simulink model "Copy_of_eCS_Algo_Simulation_2015b"  (R2015b)
settings: Solver=ode1  StartTime=0.0  StopTime=3  FixedStep=1/80000  RelTol=1e-3
PreLoadFcn:
  | if exist('tl_preloadfcn','file'), tl_preloadfcn(gcs,402); end
PostLoadFcn:
  | , if any(exist('dsrtsu_mdlpostloadfcn', 'file') == [2, 3, 6]), try dsrtsu_mdlpostloadfcn('Execute', bdroot); catch fprintf('Error in PostLoadFcn (dsrtsu_mdlpostloadfcn) for model "%s":\n %s\n', bdroot, lasterr); end, end,
  | if exist('tl_postloadfcn','file'), tl_postloadfcn(gcs,402); end
InitFcn:
  | if exist('tlds_init','file'), tlds_init(gcs); end
StartFcn:
  | if exist('tlds_start','file'), tlds_start(gcs); end
StopFcn:
  | if exist('tlds_stop','file'), tlds_stop(gcs); end
model workspace (MAT data in the model file):
  au8PrevExecProfile = [0 0 0 0 0 0]
values from neighbouring files (symbols this model uses):
  AccSensor = 5    [Parameter_eCS_Algo.m]
  AlgoType = 0    [Parameter_eCS_Algo.m]
  Cxy = 1*0.017    (= 0.017)    [Acc_Init_SelV1.m]
  Cxz = 1*0.017    (= 0.017)    [Acc_Init_SelV1.m]
  Cyx = 1*0.017    (= 0.017)    [Acc_Init_SelV1.m]
  Cyz = 1*0.017    (= 0.017)    [Acc_Init_SelV1.m]
  Czx = 1*0.017    (= 0.017)    [Acc_Init_SelV1.m]
  Czy = 1*0.017    (= 0.017)    [Acc_Init_SelV1.m]
  Forced_Oscillation = 0    [Parameter_eCS_Algo.m]    (also in run_Rotation_sim.m = run)
  FreqTemperature = 10    [Acc_Init_SelV1.m]
  MaxSensorOffset = 0.3    [Acc_Init_SelV1.m]
  Mean_x_noise = 4e-3    (= 0.004)    [Acc_Init_SelV1.m]
  Mean_y_noise = 4e-3    (= 0.004)    [Acc_Init_SelV1.m]
  Mean_z_noise = 4e-3    (= 0.004)    [Acc_Init_SelV1.m]
  ODR = 8000    [Acc_Init_SelV1.m]
  offsetcorrection_on_off = 0    [Parameter_eCS_Algo.m]
  phi_pulse_rotation = 0    [Parameter_eCS_Algo.m]    (also in run_Rotation_sim.m = angle)
  pulsetype = 2    [Parameter_eCS_Algo.m]    (also in run_simulation.m = j; run_simulation_ActiveX.m = j)
  Range = 4    [Acc_Init_SelV1.m]
  TempBias = 0    [Acc_Init_SelV1.m]
  TemperatureAmp = 0    [Acc_Init_SelV1.m]
  Var_x_noise = 1.84e-9    (= 1.84e-09)    [Acc_Init_SelV1.m]
  Var_y_noise = 2.025e-09    [Acc_Init_SelV1.m]
  Var_z_noise = 1.374e-09    [Acc_Init_SelV1.m]
  w_x = 2*pi*F_x    (= 376.991118431)    [Acc_Init_SelV1.m]
  w_y = 2*pi*F_y    (= 376.991118431)    [Acc_Init_SelV1.m]
  w_z = 2*pi*F_z    (= 376.991118431)    [Acc_Init_SelV1.m]
  x_max_temp_drift = 0.061    [Acc_Init_SelV1.m]
  x_offset_enable = 0    [Acc_Init_SelV1.m]
  x_run_to_run_drift = 0.0    (= 0)    [Acc_Init_SelV1.m]
  x_temp_co_drift = 0.000    (= 0)    [Acc_Init_SelV1.m]
  Xi_x = 0.7    [Acc_Init_SelV1.m]
  Xi_y = 0.7    [Acc_Init_SelV1.m]
  Xi_z = 0.7    [Acc_Init_SelV1.m]
  y_max_temp_drift = 0.061    [Acc_Init_SelV1.m]
  y_offset_enable = 0    [Acc_Init_SelV1.m]
  y_run_to_run_drift = 0.0    (= 0)    [Acc_Init_SelV1.m]
  y_temp_co_drift = 0.000    (= 0)    [Acc_Init_SelV1.m]
  z_max_temp_drift = 0.13    [Acc_Init_SelV1.m]
  z_offset_enable = 0    [Acc_Init_SelV1.m]
  z_run_to_run_drift = 0.0    (= 0)    [Acc_Init_SelV1.m]
  z_temp_co_drift = 0.000    (= 0)    [Acc_Init_SelV1.m]
undefined symbols (not defined in the file or in its folder): controller_sample_rate, ddv, DiscIntNeverNeededParam, ECE_L_0_x, ECE_L_0_y, ECE_L_0_z, ECE_L_45_time, ECE_L_45_x, ECE_L_45_y, ECE_L_45_z, FMVSS_45_time, FMVSS_45_x, FMVSS_45_y, FMVSS_45_z, gmw_roada_x__m_s__, gmw_roada_y__m_s__, gmw_roadtime_2kHz, KSF_50_a_x, KSF_50_a_y, KSF_50_time, KSG_30_a_x, KSG_30_a_y, KSG_30_time, Meldorf_HindenburgstraAcceleration_x__m_s_2_, Meldorf_HindenburgstraAcceleration_y__m_s_2_, Meldorf_HindenburgstraAcceleration_z__m_s_2_, Meldorf_HindenburgstraTime__s_, pulse_FF27, pulse_MPDB, pulse_ODB40, pulse_ODB64, pulse_USNCAP, pulsetime_FF27, pulsetime_MPDB, pulsetime_ODB40, pulsetime_ODB64, pulsetime_USNCAP, Rauasphalt_60_a_x, Rauasphalt_60_a_y, Rauasphalt_60_time, sigbuilder_block, TimeArray, VW_416_2kHza_x_2kHz, VW_416_2kHza_y_2kHz, VW_416_2kHztime_2kHz
libraries: simulink x40, tllib x10, tl_autosar_lib x7, simulink_extras x5, LIB_TF_G_111 x2, LIB_TF_G_12_StepControl x2, LIB_TF_G_112 x1, dspsigops x1
(part 8 of 9)

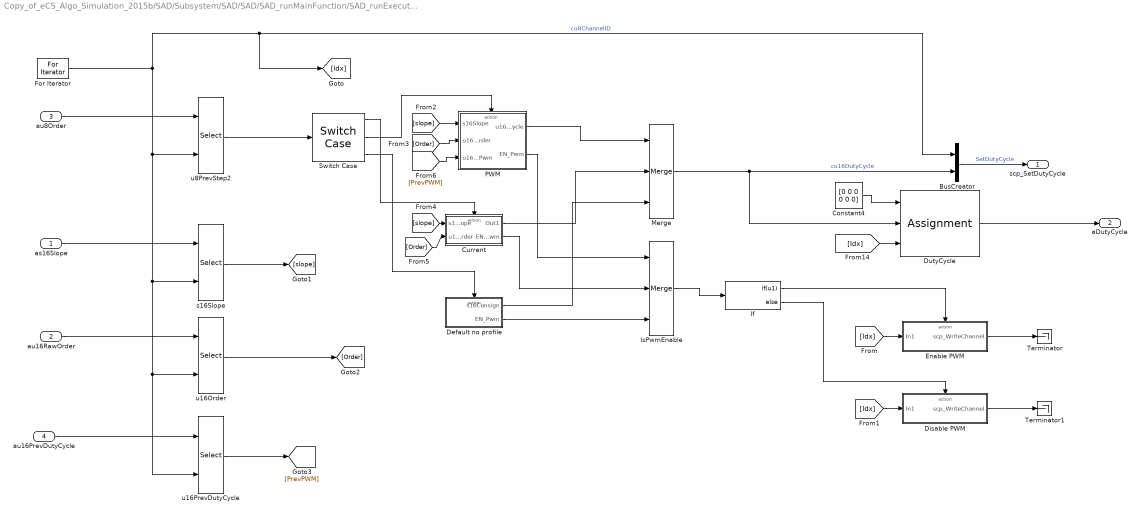
== system Copy_of_eCS_Algo_Simulation_2015b/SAD/Subsystem/SAD/SAD/SAD_runMainFunction/SAD_runExecuteStep/For Iterator Subsystem ==
  as16Slope : Inport
  au16RawOrder : Inport  Port=2
  au8Order : Inport  Port=3
  au16PrevDutyCycle : Inport  Port=4
  BusCreator : BusCreator  Inputs=2
  Constant4 : Constant  Value=[0 0 0 0 0 0]  mask(TL_Constant){data={'date',738323.57900567132}}
      settings: CopyFcn=if exist('tl_reset_reviewflag') == 2, tl_reset_reviewflag(gcbh); end  DeleteFcn=if exist('delete_tlblock','file')==2,delete_tlblock(gcbh);end  NameChangeFcn=if exist('rename_tlblock','file')==2,rename_tlblock(gcbh);end  OpenFcn=if exist('tl_open_blockdlg','file')==2,tl_open_blockdlg(gcbh);else,open_system(gcbh,'parameter');end
      mask Help: eval(['if exist(''tl_online_help'',''file'') == 2, tl_online_help(''Topic'',''TL_Constant''),else, web([''jar:file:///'',matlabroot,''/help/toolbox/simulink/help.jar!/slref/' lower(get_param(gcbh,'Blocktype')) '.html''], ''-helpbrowser''),end'])
      mask Display: plot([-0.1, 1.05, NaN, -0.1, 1.05],[.01, .01, NaN, .99, .99]);
  Current : Subsystem  TreatAsAtomicUnit=on
  Default no profile : Subsystem  TreatAsAtomicUnit=on
  Disable PWM : Subsystem  TreatAsAtomicUnit=on
  DutyCycle : Assignment  IndexMode=Zero-based  IndexOptions=Index vector (port)  Indices=1  OutputSizes=1  mask(TL_Assignment){data={'insideiteratedsystem',logical(1),'omitinitializations',1,'output',{'name','$D','type','UInt16','inheritscaling',0},'date',738370.64882278931}}
      settings: CopyFcn=if exist('tl_reset_reviewflag') == 2, tl_reset_reviewflag(gcbh); end  DeleteFcn=if exist('delete_tlblock','file')==2,delete_tlblock(gcbh);end  NameChangeFcn=if exist('rename_tlblock','file')==2,rename_tlblock(gcbh);end  OpenFcn=if exist('tl_open_blockdlg','file')==2,tl_open_blockdlg(gcbh);else,open_system(gcbh,'parameter');end
      mask Help: eval(['if exist(''tl_online_help'',''file'') == 2, tl_online_help(''Topic'',''TL_Assignment''),else, web([''jar:file:///'',matlabroot,''/help/toolbox/simulink/help.jar!/slref/' lower(get_param(gcbh,'Blocktype')) '.html''], ''-helpbrowser''),end'])
      mask Display: plot([-0.1, 1.05, NaN, -0.1, 1.05],[.01, .01, NaN, .99, .99]);
  Enable PWM : Subsystem  TreatAsAtomicUnit=on
  For Iterator : ForIterator  IterationLimit=6  IndexMode=Zero-based  IterationVariableDataType=int8
  If : If  IfExpression=u1
  IsPwmEnable : Merge  Inputs=3  mask(TL_Merge){data={'date',738338.40035140049}}
      settings: CopyFcn=if exist('tl_reset_reviewflag') == 2, tl_reset_reviewflag(gcbh); end  DeleteFcn=if exist('delete_tlblock','file')==2,delete_tlblock(gcbh);end  NameChangeFcn=if exist('rename_tlblock','file')==2,rename_tlblock(gcbh);end  OpenFcn=if exist('tl_open_blockdlg','file')==2,tl_open_blockdlg(gcbh);else,open_system(gcbh,'parameter');end
      mask Help: eval(['if exist(''tl_online_help'',''file'') == 2, tl_online_help(''Topic'',''TL_Merge''),else, web([''jar:file:///'',matlabroot,''/help/toolbox/simulink/help.jar!/slref/' lower(get_param(gcbh,'Blocktype')) '.html''], ''-helpbrowser''),end'])
      mask Display: plot([-0.1, 1.05, NaN, -0.1, 1.05],[.01, .01, NaN, .99, .99]);
  Merge : Merge  Inputs=3  mask(TL_Merge){data={'date',738338.40035140049}}
      settings: CopyFcn=if exist('tl_reset_reviewflag') == 2, tl_reset_reviewflag(gcbh); end  DeleteFcn=if exist('delete_tlblock','file')==2,delete_tlblock(gcbh);end  NameChangeFcn=if exist('rename_tlblock','file')==2,rename_tlblock(gcbh);end  OpenFcn=if exist('tl_open_blockdlg','file')==2,tl_open_blockdlg(gcbh);else,open_system(gcbh,'parameter');end
      mask Help: eval(['if exist(''tl_online_help'',''file'') == 2, tl_online_help(''Topic'',''TL_Merge''),else, web([''jar:file:///'',matlabroot,''/help/toolbox/simulink/help.jar!/slref/' lower(get_param(gcbh,'Blocktype')) '.html''], ''-helpbrowser''),end'])
      mask Display: plot([-0.1, 1.05, NaN, -0.1, 1.05],[.01, .01, NaN, .99, .99]);
  PWM : Subsystem  TreatAsAtomicUnit=on
  Switch Case : SwitchCase  CaseConditions={0,1}
  Terminator : Terminator
  Terminator1 : Terminator
  s16Slope : Selector  IndexMode=Zero-based  InputPortWidth=6  IndexOptions=Index vector (port)  Indices=[1 3]  OutputSizes=1
  u16Order : Selector  IndexMode=Zero-based  InputPortWidth=6  IndexOptions=Index vector (port)  Indices=[1 3]  OutputSizes=1
  u16PrevDutyCycle : Selector  IndexMode=Zero-based  InputPortWidth=6  IndexOptions=Index vector (port)  Indices=[1 3]  OutputSizes=1
  u8PrevStep2 : Selector  IndexMode=Zero-based  InputPortWidth=6  IndexOptions=Index vector (port)  Indices=[1 3]  OutputSizes=1
  scp_SetDutyCycle : Outport  mask(TL_BusOutport){data={'#autoscaling',2,'#message',2,'#output',2,'#logdata',2,'signals',{{'SetDutyCycle',{'cu8ChannelID';'cu16DutyCycle'}}},'autosar',{'useautosarcommunication',1,'kind',4,'clientserverport','pclPwmServices','operation','SetDutyCycle'},'date',738372.35377083335}}
      settings: CopyFcn=if exist('tl_reset_reviewflag') == 2, tl_reset_reviewflag(gcbh); end  DeleteFcn=if exist('delete_tlblock','file')==2,delete_tlblock(gcbh);end  NameChangeFcn=if exist('rename_tlblock','file')==2,rename_tlblock(gcbh);end  OpenFcn=if exist('tl_open_blockdlg','file')==2,tl_open_blockdlg(gcbh);else,open_system(gcbh,'parameter');end
      mask Help: eval(['if exist(''tl_online_help'',''file'') == 2, tl_online_help(''Topic'',''TL_Outport''),else, web([''jar:file:///'',matlabroot,''/help/toolbox/simulink/help.jar!/slref/' lower(get_param(gcbh,'Blocktype')) '.html''], ''-helpbrowser''),end'])
      mask Display: plot([0.2 0.35 NaN 0.65 0.8],[0 1 NaN 0 1]);
  aDutyCycle : Outport  Port=2
  wires:
  as16Slope/1 -> s16Slope/1
  au16RawOrder/1 -> u16Order/1
  au8Order/1 -> u8PrevStep2/1
  u8PrevStep2/1 -> Switch Case/1
  Switch Case/3 -> Default no profile/Action
  Default no profile/1(s16Consign) -> Merge/3
  Current/1(Out1) -> Merge/2
  PWM/1(u16DutyCycle) -> Merge/1
  PWM/2(EN_Pwm) -> IsPwmEnable/1
  Current/2(EN_Pwm) -> IsPwmEnable/2
  Default no profile/2(EN_Pwm) -> IsPwmEnable/3
  If/1 -> Enable PWM/Action
  IsPwmEnable/1 -> If/1
  If/2 -> Disable PWM/Action
  [Idx] -> Enable PWM/1(In1)
  [Idx] -> Disable PWM/1(In1)
  For Iterator/1 -> BusCreator/1, [Idx], s16Slope/2, u16PrevDutyCycle/2, u16Order/2, u8PrevStep2/2  "cu8ChannelID"
  Merge/1 -> DutyCycle/2, BusCreator/2  "cu16DutyCycle"
  BusCreator/1 -> scp_SetDutyCycle/1  "SetDutyCycle"
  Enable PWM/1(scp_WriteChannel) -> Terminator/1
  Disable PWM/1(scp_WriteChannel) -> Terminator1/1
  s16Slope/1 -> [slope]
  au16PrevDutyCycle/1 -> u16PrevDutyCycle/1
  u16PrevDutyCycle/1 -> [PrevPWM]
  [slope] -> PWM/1(s16Slope)
  [Order] -> PWM/2(u16RawOrder)
  [slope] -> Current/1(s16Slope)
  [Order] -> Current/2(u16RawOrder)
  DutyCycle/1 -> aDutyCycle/1
  Constant4/1 -> DutyCycle/1
  [Idx] -> DutyCycle/3
  [PrevPWM] -> PWM/3(u16PrevPwm)
  u16Order/1 -> [Order]
  Switch Case/2 -> PWM/Action
  Switch Case/1 -> Current/Action

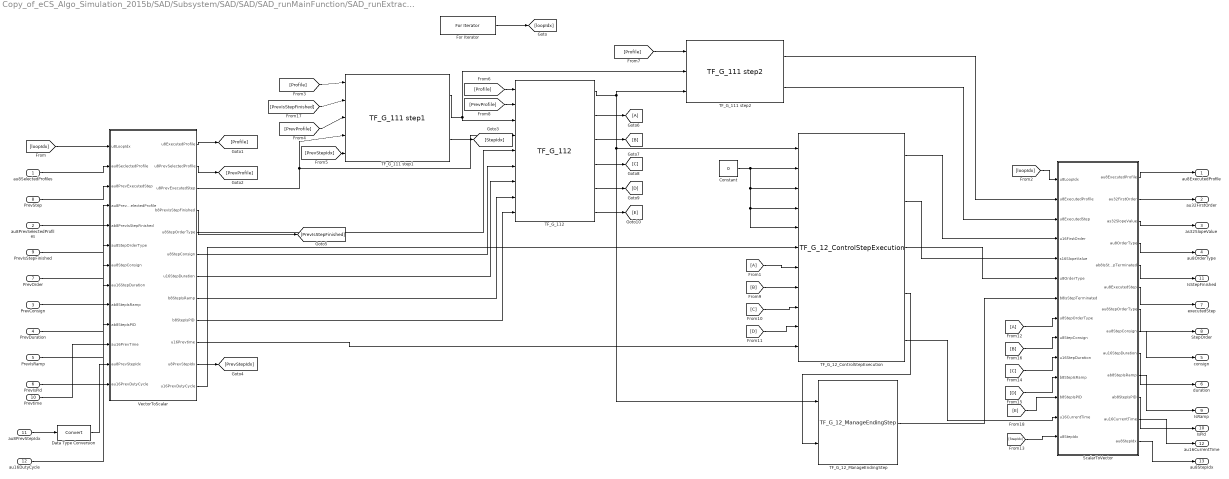
== system Copy_of_eCS_Algo_Simulation_2015b/SAD/Subsystem/SAD/SAD/SAD_runMainFunction/SAD_runExtractProfileAndStep/For Iterator Subsystem ==
  au8SelectedProfiles : Inport
  au8PrevSelectedProfiles : Inport  Port=2
  PrevConsign : Inport  Port=3
  PrevDuration : Inport  Port=4
  PrevIsRamp : Inport  Port=5
  PrevIsPid : Inport  Port=6
  PrevOrder : Inport  Port=7
  PrevStep : Inport  Port=8
  PrevIsStepFinished : Inport  Port=9
  Prevtime : Inport  Port=10
  au8PrevStepIdx : Inport  Port=11
  au16DutyCycle : Inport  Port=12
  Constant : Constant  Value=0  mask(TL_Constant){data={'date',738335.39296247682}}
      settings: CopyFcn=if exist('tl_reset_reviewflag') == 2, tl_reset_reviewflag(gcbh); end  DeleteFcn=if exist('delete_tlblock','file')==2,delete_tlblock(gcbh);end  NameChangeFcn=if exist('rename_tlblock','file')==2,rename_tlblock(gcbh);end  OpenFcn=if exist('tl_open_blockdlg','file')==2,tl_open_blockdlg(gcbh);else,open_system(gcbh,'parameter');end
      mask Help: eval(['if exist(''tl_online_help'',''file'') == 2, tl_online_help(''Topic'',''TL_Constant''),else, web([''jar:file:///'',matlabroot,''/help/toolbox/simulink/help.jar!/slref/' lower(get_param(gcbh,'Blocktype')) '.html''], ''-helpbrowser''),end'])
      mask Display: plot([-0.1, 1.05, NaN, -0.1, 1.05],[.01, .01, NaN, .99, .99]);
  Data Type Conversion : DataTypeConversion
  For Iterator : ForIterator  IterationLimit=6  IndexMode=Zero-based  IterationVariableDataType=int8
  ScalarToVector : Subsystem  TreatAsAtomicUnit=on
  TF_G_111 step1 : LIB_TF_G_111/TF_G_111 step1
  TF_G_111 step2 : LIB_TF_G_111/TF_G_111 step2  Description=The subsystemDetermineExecutedFunction block is in charge of providing the current executed function output.
  TF_G_112 : LIB_TF_G_112/TF_G_112
  TF_G_12_ControlStepExecution : LIB_TF_G_12_StepControl/TF_G_12_ControlStepExecution
  TF_G_12_ManageEndingStep : LIB_TF_G_12_StepControl/TF_G_12_ManageEndingStep
  VectorToScalar : Subsystem  TreatAsAtomicUnit=on
  au8ExecutedProfile : Outport
  au32FirstOrder : Outport  Port=2  PortDimensions=6
  as32SlopeValue : Outport  Port=3  PortDimensions=6
  au8OrderType : Outport  Port=4  PortDimensions=6
  consign : Outport  Port=5  PortDimensions=6
  duration : Outport  Port=6  PortDimensions=6
  executedStep : Outport  Port=7  PortDimensions=6
  StepOrder : Outport  Port=8  PortDimensions=6
  IsRamp : Outport  Port=9  PortDimensions=6
  IsPid : Outport  Port=10  PortDimensions=6
  IsStepFinished : Outport  Port=11  PortDimensions=6
  au16CurrentTime : Outport  Port=12  PortDimensions=6
  au8StepIdx : Outport  Port=13  PortDimensions=6
  wires:
  For Iterator/1 -> [loopIdx]
  au8SelectedProfiles/1 -> VectorToScalar/2(au8SeclectedProfile)
  [loopIdx] -> VectorToScalar/1(u8LoopIdx)
  VectorToScalar/1(u8ExecutedProfile) -> [Profile]
  VectorToScalar/2(u8PrevSelectedProfile) -> [PrevProfile]
  [Profile] -> TF_G_111 step1/1
  [PrevProfile] -> TF_G_111 step1/3
  TF_G_111 step1/1 -> TF_G_111 step2/2, TF_G_112/3
  [Profile] -> TF_G_112/1
  [Profile] -> TF_G_111 step2/1
  [PrevProfile] -> TF_G_112/2
  VectorToScalar/3(u8PrevExecutedStep) -> TF_G_111 step1/4, TF_G_112/4
  TF_G_112/1 -> TF_G_12_ControlStepExecution/1, TF_G_12_ManageEndingStep/1, TF_G_111 step2/3
  TF_G_12_ControlStepExecution/4 -> TF_G_12_ManageEndingStep/2
  ScalarToVector/6(au8ExecutedStep) -> executedStep/1
  ScalarToVector/4(au8OrderType) -> au8OrderType/1
  [PrevIsStepFinished] -> TF_G_111 step1/2
  ScalarToVector/3(as32SlopeValue) -> as32SlopeValue/1
  ScalarToVector/2(au32FirstOrder) -> au32FirstOrder/1
  ScalarToVector/1(au8ExecutedProfile) -> au8ExecutedProfile/1
  [loopIdx] -> ScalarToVector/1(u8LoopIdx)
  TF_G_111 step2/1 -> ScalarToVector/2(u8ExecutedProfile)
  TF_G_12_ControlStepExecution/2 -> ScalarToVector/5(s16SlopeValue)
  TF_G_12_ControlStepExecution/3 -> ScalarToVector/6(u8OrderType)
  TF_G_12_ManageEndingStep/1 -> ScalarToVector/7(b8IsStepTerminated)
  TF_G_111 step2/2 -> ScalarToVector/3(u8ExecutedStep)
  TF_G_112/2 -> [A]
  TF_G_112/3 -> [B]
  TF_G_112/4 -> [C]
  TF_G_112/5 -> [D]
  TF_G_112/6 -> [E]
  [A] -> TF_G_12_ControlStepExecution/7
  [C] -> TF_G_12_ControlStepExecution/9
  [D] -> TF_G_12_ControlStepExecution/10
  [A] -> ScalarToVector/8(u8StepOrderType)
  [B] -> ScalarToVector/9(u8StepConsign)
  [D] -> ScalarToVector/11(b8StepIsRamp)
  [C] -> ScalarToVector/10(u16StepDuration)
  [E] -> ScalarToVector/12(b8StepIsPID)
  ScalarToVector/8(au8StepConsign) -> consign/1
  ScalarToVector/9(au16StepDuration) -> duration/1
  VectorToScalar/5(u8StepOrderType) -> TF_G_112/5
  VectorToScalar/6(u8StepConsign) -> TF_G_112/6
  VectorToScalar/7(u16StepDuration) -> TF_G_112/7
  VectorToScalar/8(b8StepIsRamp) -> TF_G_112/8
  VectorToScalar/9(b8StepIsPID) -> TF_G_112/9
  VectorToScalar/4(b8PrevIsStepFinished) -> [PrevIsStepFinished]
  Constant/1 -> TF_G_12_ControlStepExecution/5, TF_G_12_ControlStepExecution/4, TF_G_12_ControlStepExecution/3, TF_G_12_ControlStepExecution/2
  PrevConsign/1 -> VectorToScalar/7(au8StepConsign)
  PrevDuration/1 -> VectorToScalar/8(au16StepDuration)
  ScalarToVector/11(ab8StepIsPID) -> IsPid/1
  ScalarToVector/10(ab8StepIsRamp) -> IsRamp/1
  ScalarToVector/7(au8StepOrderType) -> StepOrder/1
  PrevIsRamp/1 -> VectorToScalar/9(ab8StepIsRamp)
  PrevIsPid/1 -> VectorToScalar/10(ab8StepIsPID)
  PrevOrder/1 -> VectorToScalar/6(au8StepOrderType)
  PrevIsStepFinished/1 -> VectorToScalar/5(ab8PrevIsStepFinished)
  ScalarToVector/5(ab8IsStepTerminated) -> IsStepFinished/1
  PrevStep/1 -> VectorToScalar/3(au8PrevExecutedStep)
  au8PrevSelectedProfiles/1 -> VectorToScalar/4(au8PrevSelectedProfile)
  ScalarToVector/12(au16CurrentTime) -> au16CurrentTime/1
  TF_G_12_ControlStepExecution/5 -> ScalarToVector/13(u16CurrentTime)
  Prevtime/1 -> VectorToScalar/11(au16PrevTime)
  VectorToScalar/10(u16Prevtime) -> TF_G_12_ControlStepExecution/11
  TF_G_111 step1/2 -> [StepIdx]
  [PrevStepIdx] -> TF_G_111 step1/5
  [StepIdx] -> ScalarToVector/14(u8StepIdx)
  ScalarToVector/13(au8StepIdx) -> au8StepIdx/1
  VectorToScalar/11(u8PrevStepIdx) -> [PrevStepIdx]
  au8PrevStepIdx/1 -> Data Type Conversion/1
  Data Type Conversion/1 -> VectorToScalar/12(au8PrevStepIdx)
  [B] -> TF_G_12_ControlStepExecution/8
  TF_G_12_ControlStepExecution/1 -> ScalarToVector/4(u16FirstOrder)
  au16DutyCycle/1 -> VectorToScalar/13(au16PrevDutyCycle)
  VectorToScalar/12(u16PrevDutyCycle) -> TF_G_12_ControlStepExecution/6

== system Copy_of_eCS_Algo_Simulation_2015b/SAD/Subsystem/SAD/SAD/SAD_runMainFunction/Triggered Subsystem/If Action Subsystem ==
  Action Port : ActionPort  ActionType=then
  FcnCallGenerator : simulink/Ports & Subsystems/Function-Call Generator  sample_time=-1  numberOfIterations=1
  Out1 : Outport
  wires:
  FcnCallGenerator/1 -> Out1/1

== system Copy_of_eCS_Algo_Simulation_2015b/eCS_Targetlink/Subsystem/eCS_Targetlink/eCS_Algo_in_m_per_s-2/Crash Acceleration/Acceleration Clipping/If Action Subsystem ==
  u8Sample : Inport
  u8OldTrigger : Inport  Port=2
  u8OldTrimer : Inport  Port=3
  Action Port : ActionPort  ActionType=else
  "Clear Trigger " : Subsystem  TreatAsAtomicUnit=on
  Decrease Timer : Subsystem  TreatAsAtomicUnit=on
  If1 : If  IfExpression=u1
  Logical Operator : Logic  AllPortsSameDT=off  OutDataTypeStr=boolean  mask(TL_LogicalOperator){data={'date',738071.59304812504}}
      settings: DeleteFcn=if exist('delete_tlblock','file')==2,delete_tlblock(gcbh);end  NameChangeFcn=if exist('rename_tlblock','file')==2,rename_tlblock(gcbh);end  OpenFcn=if exist('tl_open_blockdlg','file')==2,tl_open_blockdlg(gcbh);else,open_system(gcbh,'parameter');end
      mask Help: eval(['if exist(''tl_online_help'',''file'') == 2, tl_online_help(''Topic'',''TL_LogicalOperator''),else, web([''jar:file:///'',matlabroot,''/help/toolbox/simulink/help.jar!/slref/' lower(get_param(gcbh,'Blocktype')) '.html''], ''-helpbrowser''),end'])
      mask Display: plot([-0.1, 1.05, NaN, -0.1, 1.05],[.01, .01, NaN, .99, .99]);
  Logical Operator1 : Logic  AllPortsSameDT=off  OutDataTypeStr=boolean  mask(TL_LogicalOperator){data={'date',738071.59304820606}}
      settings: DeleteFcn=if exist('delete_tlblock','file')==2,delete_tlblock(gcbh);end  NameChangeFcn=if exist('rename_tlblock','file')==2,rename_tlblock(gcbh);end  OpenFcn=if exist('tl_open_blockdlg','file')==2,tl_open_blockdlg(gcbh);else,open_system(gcbh,'parameter');end
      mask Help: eval(['if exist(''tl_online_help'',''file'') == 2, tl_online_help(''Topic'',''TL_LogicalOperator''),else, web([''jar:file:///'',matlabroot,''/help/toolbox/simulink/help.jar!/slref/' lower(get_param(gcbh,'Blocktype')) '.html''], ''-helpbrowser''),end'])
      mask Display: plot([-0.1, 1.05, NaN, -0.1, 1.05],[.01, .01, NaN, .99, .99]);
  MaxSample2 : Constant  Value=ddv('eCS_CFG/CRASH_SAMPLES_NB')  mask(TL_Constant){data={'output',{'variable','eCS_CFG/CRASH_SAMPLES_NB'},'date',738071.59304828709}}
      settings: CopyFcn=if exist('tl_reset_reviewflag') == 2, tl_reset_reviewflag(gcbh); end  DeleteFcn=if exist('delete_tlblock','file')==2,delete_tlblock(gcbh);end  NameChangeFcn=if exist('rename_tlblock','file')==2,rename_tlblock(gcbh);end  OpenFcn=if exist('tl_open_blockdlg','file')==2,tl_open_blockdlg(gcbh);else,open_system(gcbh,'parameter');end
      mask Help: eval(['if exist(''tl_online_help'',''file'') == 2, tl_online_help(''Topic'',''TL_Constant''),else, web([''jar:file:///'',matlabroot,''/help/toolbox/simulink/help.jar!/slref/' lower(get_param(gcbh,'Blocktype')) '.html''], ''-helpbrowser''),end'])
      mask Display: plot([-0.1, 1.05, NaN, -0.1, 1.05],[.01, .01, NaN, .99, .99]);
  MaxSample3 : Constant  mask(TL_Constant){data={'date',738071.593048368}}
      settings: CopyFcn=if exist('tl_reset_reviewflag') == 2, tl_reset_reviewflag(gcbh); end  DeleteFcn=if exist('delete_tlblock','file')==2,delete_tlblock(gcbh);end  NameChangeFcn=if exist('rename_tlblock','file')==2,rename_tlblock(gcbh);end  OpenFcn=if exist('tl_open_blockdlg','file')==2,tl_open_blockdlg(gcbh);else,open_system(gcbh,'parameter');end
      mask Help: eval(['if exist(''tl_online_help'',''file'') == 2, tl_online_help(''Topic'',''TL_Constant''),else, web([''jar:file:///'',matlabroot,''/help/toolbox/simulink/help.jar!/slref/' lower(get_param(gcbh,'Blocktype')) '.html''], ''-helpbrowser''),end'])
      mask Display: plot([-0.1, 1.05, NaN, -0.1, 1.05],[.01, .01, NaN, .99, .99]);
  MaxSample4 : Constant  Value=0  mask(TL_Constant){data={'date',738071.59304844902}}
      settings: CopyFcn=if exist('tl_reset_reviewflag') == 2, tl_reset_reviewflag(gcbh); end  DeleteFcn=if exist('delete_tlblock','file')==2,delete_tlblock(gcbh);end  NameChangeFcn=if exist('rename_tlblock','file')==2,rename_tlblock(gcbh);end  OpenFcn=if exist('tl_open_blockdlg','file')==2,tl_open_blockdlg(gcbh);else,open_system(gcbh,'parameter');end
      mask Help: eval(['if exist(''tl_online_help'',''file'') == 2, tl_online_help(''Topic'',''TL_Constant''),else, web([''jar:file:///'',matlabroot,''/help/toolbox/simulink/help.jar!/slref/' lower(get_param(gcbh,'Blocktype')) '.html''], ''-helpbrowser''),end'])
      mask Display: plot([-0.1, 1.05, NaN, -0.1, 1.05],[.01, .01, NaN, .99, .99]);
  Merge : Merge  InitialOutput=0  mask(TL_Merge){data={'date',738071.59304854169}}
      settings: CopyFcn=if exist('tl_reset_reviewflag') == 2, tl_reset_reviewflag(gcbh); end  DeleteFcn=if exist('delete_tlblock','file')==2,delete_tlblock(gcbh);end  NameChangeFcn=if exist('rename_tlblock','file')==2,rename_tlblock(gcbh);end  OpenFcn=if exist('tl_open_blockdlg','file')==2,tl_open_blockdlg(gcbh);else,open_system(gcbh,'parameter');end
      mask Help: eval(['if exist(''tl_online_help'',''file'') == 2, tl_online_help(''Topic'',''TL_Merge''),else, web([''jar:file:///'',matlabroot,''/help/toolbox/simulink/help.jar!/slref/' lower(get_param(gcbh,'Blocktype')) '.html''], ''-helpbrowser''),end'])
      mask Display: plot([-0.1, 1.05, NaN, -0.1, 1.05],[.01, .01, NaN, .99, .99]);
  Merge1 : Merge  InitialOutput=0  mask(TL_Merge){data={'date',738071.59304862272}}
      settings: CopyFcn=if exist('tl_reset_reviewflag') == 2, tl_reset_reviewflag(gcbh); end  DeleteFcn=if exist('delete_tlblock','file')==2,delete_tlblock(gcbh);end  NameChangeFcn=if exist('rename_tlblock','file')==2,rename_tlblock(gcbh);end  OpenFcn=if exist('tl_open_blockdlg','file')==2,tl_open_blockdlg(gcbh);else,open_system(gcbh,'parameter');end
      mask Help: eval(['if exist(''tl_online_help'',''file'') == 2, tl_online_help(''Topic'',''TL_Merge''),else, web([''jar:file:///'',matlabroot,''/help/toolbox/simulink/help.jar!/slref/' lower(get_param(gcbh,'Blocktype')) '.html''], ''-helpbrowser''),end'])
      mask Display: plot([-0.1, 1.05, NaN, -0.1, 1.05],[.01, .01, NaN, .99, .99]);
  Relational Operator2 : RelationalOperator  Operator=<  OutDataTypeStr=boolean  mask(TL_RelationalOperator){data={'date',738071.59304870374}}
      settings: DeleteFcn=if exist('delete_tlblock','file')==2,delete_tlblock(gcbh);end  NameChangeFcn=if exist('rename_tlblock','file')==2,rename_tlblock(gcbh);end  OpenFcn=if exist('tl_open_blockdlg','file')==2,tl_open_blockdlg(gcbh);else,open_system(gcbh,'parameter');end
      mask Help: eval(['if exist(''tl_online_help'',''file'') == 2, tl_online_help(''Topic'',''TL_RelationalOperator''),else, web([''jar:file:///'',matlabroot,''/help/toolbox/simulink/help.jar!/slref/' lower(get_param(gcbh,'Blocktype')) '.html''], ''-helpbrowser''),end'])
      mask Display: plot([-0.1, 1.05, NaN, -0.1, 1.05],[.01, .01, NaN, .99, .99]);
  Relational Operator3 : RelationalOperator  Operator===  OutDataTypeStr=boolean  mask(TL_RelationalOperator){data={'date',738071.59304878477}}
      settings: DeleteFcn=if exist('delete_tlblock','file')==2,delete_tlblock(gcbh);end  NameChangeFcn=if exist('rename_tlblock','file')==2,rename_tlblock(gcbh);end  OpenFcn=if exist('tl_open_blockdlg','file')==2,tl_open_blockdlg(gcbh);else,open_system(gcbh,'parameter');end
      mask Help: eval(['if exist(''tl_online_help'',''file'') == 2, tl_online_help(''Topic'',''TL_RelationalOperator''),else, web([''jar:file:///'',matlabroot,''/help/toolbox/simulink/help.jar!/slref/' lower(get_param(gcbh,'Blocktype')) '.html''], ''-helpbrowser''),end'])
      mask Display: plot([-0.1, 1.05, NaN, -0.1, 1.05],[.01, .01, NaN, .99, .99]);
  Relational Operator4 : RelationalOperator  Operator===  OutDataTypeStr=boolean  mask(TL_RelationalOperator){data={'date',738071.59304885415}}
      settings: DeleteFcn=if exist('delete_tlblock','file')==2,delete_tlblock(gcbh);end  NameChangeFcn=if exist('rename_tlblock','file')==2,rename_tlblock(gcbh);end  OpenFcn=if exist('tl_open_blockdlg','file')==2,tl_open_blockdlg(gcbh);else,open_system(gcbh,'parameter');end
      mask Help: eval(['if exist(''tl_online_help'',''file'') == 2, tl_online_help(''Topic'',''TL_RelationalOperator''),else, web([''jar:file:///'',matlabroot,''/help/toolbox/simulink/help.jar!/slref/' lower(get_param(gcbh,'Blocktype')) '.html''], ''-helpbrowser''),end'])
      mask Display: plot([-0.1, 1.05, NaN, -0.1, 1.05],[.01, .01, NaN, .99, .99]);
  u8Trigger : Outport  InitialOutput=0
  u16Timer : Outport  Port=2  InitialOutput=0
  wires:
  If1/1 -> "Clear Trigger "/Action
  u8Sample/1 -> Relational Operator2/1
  MaxSample2/1 -> Relational Operator2/2
  u8OldTrigger/1 -> Decrease Timer/2(u8OldTrigger), Relational Operator3/2
  MaxSample3/1 -> Relational Operator3/1
  MaxSample4/1 -> Relational Operator4/2
  Relational Operator2/1 -> Logical Operator/1
  Relational Operator3/1 -> Logical Operator/2
  Relational Operator4/1 -> Logical Operator1/2
  Logical Operator/1 -> Logical Operator1/1
  Logical Operator1/1 -> If1/1
  If1/2 -> Decrease Timer/Action
  u8OldTrimer/1 -> "Clear Trigger "/1(u16OldTimer), Relational Operator4/1, Decrease Timer/1(u16OldTimer)
  Merge/1 -> u8Trigger/1
  "Clear Trigger "/1(Trigger) -> Merge/1
  Merge1/1 -> u16Timer/1
  Decrease Timer/1(u16Timer) -> Merge1/1
  Decrease Timer/2(Trigger) -> Merge/2
  "Clear Trigger "/2(u16Timer) -> Merge1/2

== system Copy_of_eCS_Algo_Simulation_2015b/eCS_Targetlink/Subsystem/eCS_Targetlink/eCS_Algo_in_m_per_s-2/Crash Acceleration/Acceleration Clipping/Reset timer ==
  Action Port : ActionPort  ActionType=then
  HoldingTime : Constant  Value=ddv('eCS_CFG/CRASH_HOLDING_TMR')  mask(TL_Constant){data={'output',{'variable','eCS_CFG/CRASH_HOLDING_TMR'},'date',738071.59304978012}}
      settings: CopyFcn=if exist('tl_reset_reviewflag') == 2, tl_reset_reviewflag(gcbh); end  DeleteFcn=if exist('delete_tlblock','file')==2,delete_tlblock(gcbh);end  NameChangeFcn=if exist('rename_tlblock','file')==2,rename_tlblock(gcbh);end  OpenFcn=if exist('tl_open_blockdlg','file')==2,tl_open_blockdlg(gcbh);else,open_system(gcbh,'parameter');end
      mask Help: eval(['if exist(''tl_online_help'',''file'') == 2, tl_online_help(''Topic'',''TL_Constant''),else, web([''jar:file:///'',matlabroot,''/help/toolbox/simulink/help.jar!/slref/' lower(get_param(gcbh,'Blocktype')) '.html''], ''-helpbrowser''),end'])
      mask Display: plot([-0.1, 1.05, NaN, -0.1, 1.05],[.01, .01, NaN, .99, .99]);
  HoldingTime1 : Constant  mask(TL_Constant){data={'date',738071.59304987267}}
      settings: CopyFcn=if exist('tl_reset_reviewflag') == 2, tl_reset_reviewflag(gcbh); end  DeleteFcn=if exist('delete_tlblock','file')==2,delete_tlblock(gcbh);end  NameChangeFcn=if exist('rename_tlblock','file')==2,rename_tlblock(gcbh);end  OpenFcn=if exist('tl_open_blockdlg','file')==2,tl_open_blockdlg(gcbh);else,open_system(gcbh,'parameter');end
      mask Help: eval(['if exist(''tl_online_help'',''file'') == 2, tl_online_help(''Topic'',''TL_Constant''),else, web([''jar:file:///'',matlabroot,''/help/toolbox/simulink/help.jar!/slref/' lower(get_param(gcbh,'Blocktype')) '.html''], ''-helpbrowser''),end'])
      mask Display: plot([-0.1, 1.05, NaN, -0.1, 1.05],[.01, .01, NaN, .99, .99]);
  u16Timer : Outport  InitialOutput=0
  u8Trigger : Outport  Port=2  InitialOutput=1
  wires:
  HoldingTime/1 -> u16Timer/1
  HoldingTime1/1 -> u8Trigger/1

== system Copy_of_eCS_Algo_Simulation_2015b/SAD/Subsystem/SAD/SAD/SAD_runMainFunction/SAD_runExecuteStep/For Iterator Subsystem/Current ==
  s16Slope : Inport
  u16RawOrder : Inport  Port=2
  Action Port : ActionPort  ActionType=case
  Constant : Constant  Value=ddv('Common/KU8_ONE')  mask(TL_Constant){data={'output',{'variable','Common/KU8_ONE'},'date',738338.41043023148}}
      settings: CopyFcn=if exist('tl_reset_reviewflag') == 2, tl_reset_reviewflag(gcbh); end  DeleteFcn=if exist('delete_tlblock','file')==2,delete_tlblock(gcbh);end  NameChangeFcn=if exist('rename_tlblock','file')==2,rename_tlblock(gcbh);end  OpenFcn=if exist('tl_open_blockdlg','file')==2,tl_open_blockdlg(gcbh);else,open_system(gcbh,'parameter');end
      mask Help: eval(['if exist(''tl_online_help'',''file'') == 2, tl_online_help(''Topic'',''TL_Constant''),else, web([''jar:file:///'',matlabroot,''/help/toolbox/simulink/help.jar!/slref/' lower(get_param(gcbh,'Blocktype')) '.html''], ''-helpbrowser''),end'])
      mask Display: plot([-0.1, 1.05, NaN, -0.1, 1.05],[.01, .01, NaN, .99, .99]);
  Out1 : Outport
  EN_Pwm : Outport  Port=2
  wires:
  Constant/1 -> EN_Pwm/1
  u16RawOrder/1 -> Out1/1

== system Copy_of_eCS_Algo_Simulation_2015b/SAD/Subsystem/SAD/SAD/SAD_runMainFunction/SAD_runExecuteStep/For Iterator Subsystem/Default no profile ==
  Action Port : ActionPort  ActionType=default
  Constant : Constant  Value=ddv('Common/KU16_ZERO')  mask(TL_Constant){data={'output',{'variable','Common/KU16_ZERO'},'date',738370.65443438652}}
      settings: CopyFcn=if exist('tl_reset_reviewflag') == 2, tl_reset_reviewflag(gcbh); end  DeleteFcn=if exist('delete_tlblock','file')==2,delete_tlblock(gcbh);end  NameChangeFcn=if exist('rename_tlblock','file')==2,rename_tlblock(gcbh);end  OpenFcn=if exist('tl_open_blockdlg','file')==2,tl_open_blockdlg(gcbh);else,open_system(gcbh,'parameter');end
      mask Help: eval(['if exist(''tl_online_help'',''file'') == 2, tl_online_help(''Topic'',''TL_Constant''),else, web([''jar:file:///'',matlabroot,''/help/toolbox/simulink/help.jar!/slref/' lower(get_param(gcbh,'Blocktype')) '.html''], ''-helpbrowser''),end'])
      mask Display: plot([-0.1, 1.05, NaN, -0.1, 1.05],[.01, .01, NaN, .99, .99]);
  Constant1 : Constant  Value=ddv('Common/KU8_ZERO')  mask(TL_Constant){data={'output',{'variable','Common/KU8_ZERO'},'date',738338.41029982641}}
      settings: CopyFcn=if exist('tl_reset_reviewflag') == 2, tl_reset_reviewflag(gcbh); end  DeleteFcn=if exist('delete_tlblock','file')==2,delete_tlblock(gcbh);end  NameChangeFcn=if exist('rename_tlblock','file')==2,rename_tlblock(gcbh);end  OpenFcn=if exist('tl_open_blockdlg','file')==2,tl_open_blockdlg(gcbh);else,open_system(gcbh,'parameter');end
      mask Help: eval(['if exist(''tl_online_help'',''file'') == 2, tl_online_help(''Topic'',''TL_Constant''),else, web([''jar:file:///'',matlabroot,''/help/toolbox/simulink/help.jar!/slref/' lower(get_param(gcbh,'Blocktype')) '.html''], ''-helpbrowser''),end'])
      mask Display: plot([-0.1, 1.05, NaN, -0.1, 1.05],[.01, .01, NaN, .99, .99]);
  s16Consign : Outport
  EN_Pwm : Outport  Port=2
  wires:
  Constant/1 -> s16Consign/1
  Constant1/1 -> EN_Pwm/1

== system Copy_of_eCS_Algo_Simulation_2015b/SAD/Subsystem/SAD/SAD/SAD_runMainFunction/SAD_runExecuteStep/For Iterator Subsystem/Disable PWM ==
  In1 : Inport
  Action Port : ActionPort  ActionType=else
  BusCreator : BusCreator  Inputs=2
  Constant : Constant  Value=ddv('Common/KU8_ZERO')  mask(TL_Constant){data={'output',{'variable','Common/KU8_ZERO'},'date',738339.44965553237}}
      settings: CopyFcn=if exist('tl_reset_reviewflag') == 2, tl_reset_reviewflag(gcbh); end  DeleteFcn=if exist('delete_tlblock','file')==2,delete_tlblock(gcbh);end  NameChangeFcn=if exist('rename_tlblock','file')==2,rename_tlblock(gcbh);end  OpenFcn=if exist('tl_open_blockdlg','file')==2,tl_open_blockdlg(gcbh);else,open_system(gcbh,'parameter');end
      mask Help: eval(['if exist(''tl_online_help'',''file'') == 2, tl_online_help(''Topic'',''TL_Constant''),else, web([''jar:file:///'',matlabroot,''/help/toolbox/simulink/help.jar!/slref/' lower(get_param(gcbh,'Blocktype')) '.html''], ''-helpbrowser''),end'])
      mask Display: plot([-0.1, 1.05, NaN, -0.1, 1.05],[.01, .01, NaN, .99, .99]);
  scp_WriteChannel : Outport  mask(TL_BusOutport){data={'#autoscaling',2,'#message',2,'#output',2,'#logdata',2,'signals',{{'WriteChannel',{'u8ChannelID';'u8Level'}}},'autosar',{'useautosarcommunication',1,'kind',4,'clientserverport','pclDioIfServices','operation','WriteChannel'},'date',738339.44715271995}}
      settings: CopyFcn=if exist('tl_reset_reviewflag') == 2, tl_reset_reviewflag(gcbh); end  DeleteFcn=if exist('delete_tlblock','file')==2,delete_tlblock(gcbh);end  NameChangeFcn=if exist('rename_tlblock','file')==2,rename_tlblock(gcbh);end  OpenFcn=if exist('tl_open_blockdlg','file')==2,tl_open_blockdlg(gcbh);else,open_system(gcbh,'parameter');end
      mask Help: eval(['if exist(''tl_online_help'',''file'') == 2, tl_online_help(''Topic'',''TL_Outport''),else, web([''jar:file:///'',matlabroot,''/help/toolbox/simulink/help.jar!/slref/' lower(get_param(gcbh,'Blocktype')) '.html''], ''-helpbrowser''),end'])
      mask Display: plot([0.2 0.35 NaN 0.65 0.8],[0 1 NaN 0 1]);
  wires:
  In1/1 -> BusCreator/1  "u8ChannelID"
  Constant/1 -> BusCreator/2  "u8Level"
  BusCreator/1 -> scp_WriteChannel/1  "WriteChannel"

== system Copy_of_eCS_Algo_Simulation_2015b/SAD/Subsystem/SAD/SAD/SAD_runMainFunction/SAD_runExecuteStep/For Iterator Subsystem/Enable PWM ==
  In1 : Inport
  Action Port : ActionPort  ActionType=then
  BusCreator : BusCreator  Inputs=2
  Constant : Constant  Value=ddv('Common/KU8_ONE')  mask(TL_Constant){data={'output',{'variable','Common/KU8_ONE'},'date',738339.44936673611}}
      settings: CopyFcn=if exist('tl_reset_reviewflag') == 2, tl_reset_reviewflag(gcbh); end  DeleteFcn=if exist('delete_tlblock','file')==2,delete_tlblock(gcbh);end  NameChangeFcn=if exist('rename_tlblock','file')==2,rename_tlblock(gcbh);end  OpenFcn=if exist('tl_open_blockdlg','file')==2,tl_open_blockdlg(gcbh);else,open_system(gcbh,'parameter');end
      mask Help: eval(['if exist(''tl_online_help'',''file'') == 2, tl_online_help(''Topic'',''TL_Constant''),else, web([''jar:file:///'',matlabroot,''/help/toolbox/simulink/help.jar!/slref/' lower(get_param(gcbh,'Blocktype')) '.html''], ''-helpbrowser''),end'])
      mask Display: plot([-0.1, 1.05, NaN, -0.1, 1.05],[.01, .01, NaN, .99, .99]);
  scp_WriteChannel : Outport  mask(TL_BusOutport){data={'#autoscaling',2,'#message',2,'#output',2,'#logdata',2,'signals',{{'WriteChannel',{'u8ChannelID';'u8Level'}}},'autosar',{'useautosarcommunication',1,'kind',4,'clientserverport','pclDioIfServices','operation','WriteChannel'},'date',738339.44715271995}}
      settings: CopyFcn=if exist('tl_reset_reviewflag') == 2, tl_reset_reviewflag(gcbh); end  DeleteFcn=if exist('delete_tlblock','file')==2,delete_tlblock(gcbh);end  NameChangeFcn=if exist('rename_tlblock','file')==2,rename_tlblock(gcbh);end  OpenFcn=if exist('tl_open_blockdlg','file')==2,tl_open_blockdlg(gcbh);else,open_system(gcbh,'parameter');end
      mask Help: eval(['if exist(''tl_online_help'',''file'') == 2, tl_online_help(''Topic'',''TL_Outport''),else, web([''jar:file:///'',matlabroot,''/help/toolbox/simulink/help.jar!/slref/' lower(get_param(gcbh,'Blocktype')) '.html''], ''-helpbrowser''),end'])
      mask Display: plot([0.2 0.35 NaN 0.65 0.8],[0 1 NaN 0 1]);
  wires:
  In1/1 -> BusCreator/1  "u8ChannelID"
  Constant/1 -> BusCreator/2  "u8Level"
  BusCreator/1 -> scp_WriteChannel/1  "WriteChannel"

== system Copy_of_eCS_Algo_Simulation_2015b/SAD/Subsystem/SAD/SAD/SAD_runMainFunction/SAD_runExecuteStep/For Iterator Subsystem/PWM ==
  s16Slope : Inport
  u16RawOrder : Inport  Port=2
  u16PrevPwm : Inport  Port=3
  Action Port : ActionPort  ActionType=case
  Constant : Constant  Value=ddv('Common/KU8_ONE')  mask(TL_Constant){data={'output',{'variable','Common/KU8_ONE'},'date',738338.41050665511}}
      settings: CopyFcn=if exist('tl_reset_reviewflag') == 2, tl_reset_reviewflag(gcbh); end  DeleteFcn=if exist('delete_tlblock','file')==2,delete_tlblock(gcbh);end  NameChangeFcn=if exist('rename_tlblock','file')==2,rename_tlblock(gcbh);end  OpenFcn=if exist('tl_open_blockdlg','file')==2,tl_open_blockdlg(gcbh);else,open_system(gcbh,'parameter');end
      mask Help: eval(['if exist(''tl_online_help'',''file'') == 2, tl_online_help(''Topic'',''TL_Constant''),else, web([''jar:file:///'',matlabroot,''/help/toolbox/simulink/help.jar!/slref/' lower(get_param(gcbh,'Blocktype')) '.html''], ''-helpbrowser''),end'])
      mask Display: plot([-0.1, 1.05, NaN, -0.1, 1.05],[.01, .01, NaN, .99, .99]);
  Ramp : Switch  Criteria=u2 ~= 0  mask(TL_Switch){data={'output',{'type','UInt16'},'date',738372.36244082171}}
      settings: CopyFcn=if exist('tl_reset_reviewflag') == 2, tl_reset_reviewflag(gcbh); end  DeleteFcn=if exist('delete_tlblock','file')==2,delete_tlblock(gcbh);end  NameChangeFcn=if exist('rename_tlblock','file')==2,rename_tlblock(gcbh);end  OpenFcn=if exist('tl_open_blockdlg','file')==2,tl_open_blockdlg(gcbh);else,open_system(gcbh,'parameter');end
      mask Help: eval(['if exist(''tl_online_help'',''file'') == 2, tl_online_help(''Topic'',''TL_Switch''),else, web([''jar:file:///'',matlabroot,''/help/toolbox/simulink/help.jar!/slref/' lower(get_param(gcbh,'Blocktype')) '.html''], ''-helpbrowser''),end'])
      mask Display: plot([-0.1, 1.05, NaN, -0.1, 1.05],[.01, .01, NaN, .99, .99]);
  Sum : Sum  mask(TL_Sum){data={'output',{'type','UInt16'},'date',738372.36090223375}}
      settings: CopyFcn=if exist('tl_reset_reviewflag') == 2, tl_reset_reviewflag(gcbh); end  DeleteFcn=if exist('delete_tlblock','file')==2,delete_tlblock(gcbh);end  NameChangeFcn=if exist('rename_tlblock','file')==2,rename_tlblock(gcbh);end  OpenFcn=if exist('tl_open_blockdlg','file')==2,tl_open_blockdlg(gcbh);else,open_system(gcbh,'parameter');end
      mask Help: eval(['if exist(''tl_online_help'',''file'') == 2, tl_online_help(''Topic'',''TL_Sum''),else, web([''jar:file:///'',matlabroot,''/help/toolbox/simulink/help.jar!/slref/' lower(get_param(gcbh,'Blocktype')) '.html''], ''-helpbrowser''),end'])
      mask Display: plot([-0.1, 1.05, NaN, -0.1, 1.05],[.01, .01, NaN, .99, .99]);
  u16DutyCycle : Outport
  EN_Pwm : Outport  Port=2
  wires:
  Constant/1 -> EN_Pwm/1
  u16RawOrder/1 -> Ramp/3
  Sum/1 -> Ramp/1
  Ramp/1 -> u16DutyCycle/1
  u16PrevPwm/1 -> Sum/1
  s16Slope/1 -> Sum/2, Ramp/2
